simulink model "two_phase_salient_electric_machine"  (R2017b)
settings: Solver=VariableStepAuto  StartTime=0.0  StopTime=100  RelTol=1e-3
values from neighbouring files (symbols this model uses):
  dLm = 1    [two_phase_salient_electric_machine_parameters.m]
  dLr = 4    [two_phase_salient_electric_machine_parameters.m]
  dLs = 4    [two_phase_salient_electric_machine_parameters.m]
  J = 1    [two_phase_salient_electric_machine_parameters.m]
  Lm = 2    [two_phase_salient_electric_machine_parameters.m]
  Lr = 10    [two_phase_salient_electric_machine_parameters.m]
  Ls = 10    [two_phase_salient_electric_machine_parameters.m]
  Rrd = 10    [two_phase_salient_electric_machine_parameters.m]
  Rrq = 10    [two_phase_salient_electric_machine_parameters.m]
  Rsa = 10    [two_phase_salient_electric_machine_parameters.m]
  Rsb = 10    [two_phase_salient_electric_machine_parameters.m]
settings Model: Creator=Алексей  LastModifiedBy=Алексей

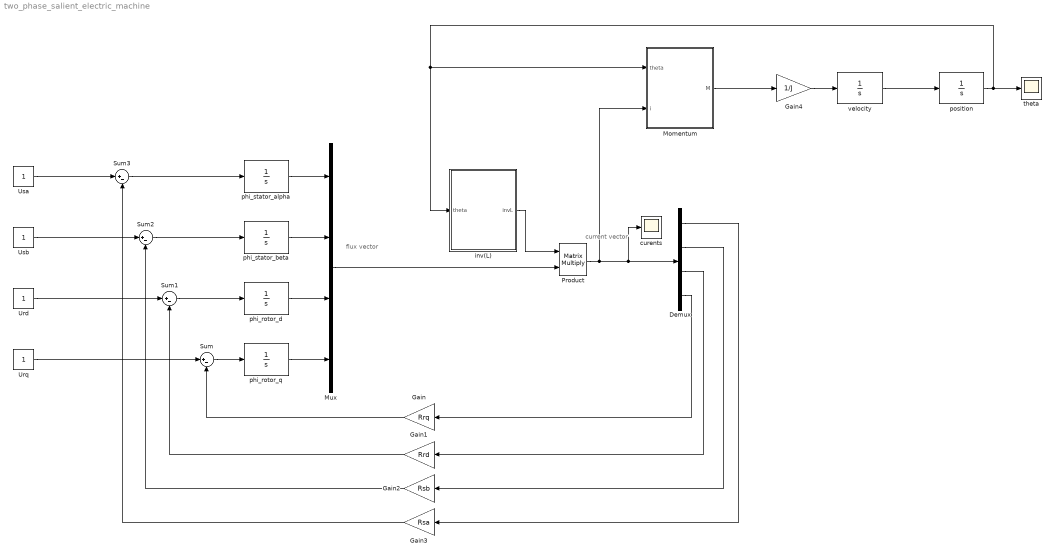
== system two_phase_salient_electric_machine ==
  note: current vector
  note: flux vector
  Demux : Demux
  Gain : Gain  Gain=Rrq
  Gain1 : Gain  Gain=Rrd
  Gain2 : Gain  Gain=Rsb
  Gain3 : Gain  Gain=Rsa
  Gain4 : Gain  Gain=1/J
  Momentum : MATLAB Function  TreatAsAtomicUnit=on
  Mux : Mux
  Product : Product  Multiplication=Matrix(*)
  Sum{,1..3} (4 alike) : Sum  Inputs=|+-
  Urd : Constant
  Urq : Constant
  Usa : Constant
  Usb : Constant
  curents : Scope
  inv(L) : MATLAB Function  TreatAsAtomicUnit=on
  phi_rotor_d : Integrator
  phi_rotor_q : Integrator
  phi_stator_alpha : Integrator
  phi_stator_beta : Integrator
  position : Integrator
  theta : Scope
  velocity : Integrator
  wires:
  velocity/1 -> position/1
  phi_stator_alpha/1 -> Mux/1
  phi_stator_beta/1 -> Mux/2
  phi_rotor_d/1 -> Mux/3
  phi_rotor_q/1 -> Mux/4
  inv(L)/1(invL) -> Product/1
  Mux/1 -> Product/2
  Product/1 -> Momentum/2(i), curents/1, Demux/1
  Sum/1 -> phi_rotor_q/1
  Demux/4 -> Gain/1
  Gain/1 -> Sum/2
  Sum1/1 -> phi_rotor_d/1
  Demux/3 -> Gain1/1
  Gain1/1 -> Sum1/2
  Demux/2 -> Gain2/1
  Demux/1 -> Gain3/1
  Gain2/1 -> Sum2/2
  Gain3/1 -> Sum3/2
  Sum2/1 -> phi_stator_beta/1
  Sum3/1 -> phi_stator_alpha/1
  Urq/1 -> Sum/1
  Urd/1 -> Sum1/1
  Usb/1 -> Sum2/1
  Usa/1 -> Sum3/1
  Gain4/1 -> velocity/1
  Momentum/1(M) -> Gain4/1
  position/1 -> theta/1, Momentum/1(theta), inv(L)/1(theta)

== matlab function two_phase_salient_electric_machine/Momentum ==
  data: theta input; i input size=4; M output; Lm parameter; dLm parameter
function M = M_calc(theta, i, Lm, dLm)
i_sa = i(1);
i_sb = i(2);
i_rd = i(3);
i_rq = i(4);
M =-i_sa*i_rd*(Lm+dLm)*sin(theta)...
    -i_sa*i_rq*(Lm-dLm)*cos(theta)...
    +i_sb*i_rd*(Lm+dLm)*cos(theta)...
    -i_sb*i_rq*(Lm-dLm)*sin(theta);

== matlab function two_phase_salient_electric_machine/inv(L) ==
  data: theta input; invL output size=[4,4]; Ls parameter; dLs parameter; Lm parameter; dLm parameter; Lr parameter; dLr parameter
function invL = invL_calc(theta, Ls, dLs, Lm, dLm, Lr, dLr)

L = [Ls+dLs*cos(2*theta)  dLs*sin(2*theta)  (Lm+dLm)*cos(theta)  -(Lm-dLm)*sin(theta);
     dLs*sin(2*theta)  Ls-dLs*cos(2*theta)  (Lm+dLm)*sin(theta)  (Lm-dLm)*cos(theta);
     (Lm+dLm)*cos(theta)  (Lm+dLm)*sin(theta)  Lr+dLr, 0;
     -(Lm-dLm)*sin(theta)  (Lm-dLm)*cos(theta)  0  Lr-dLr];
invL = inv(L);
